simulink model "module_12s"  (R2024b)
settings: Solver=ode4  StartTime=0.0  StopTime=T_stop  FixedStep=0.1  RelTol=1e-3
settings Model: Creator=rayen  LastModifiedBy=dhia
settings DebuggingCC: AlgebraicLoopMsg=none

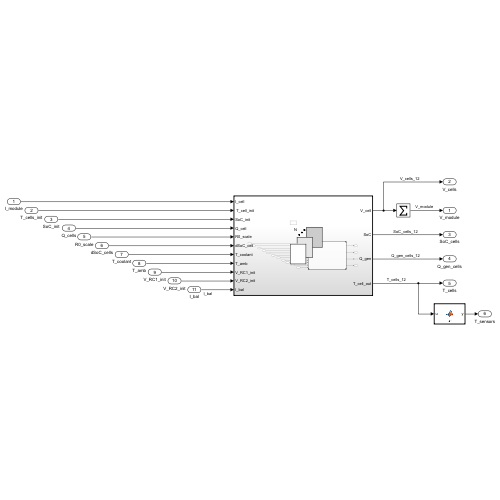
[thumbnail: Simulink's stored preview of the top-level diagram]
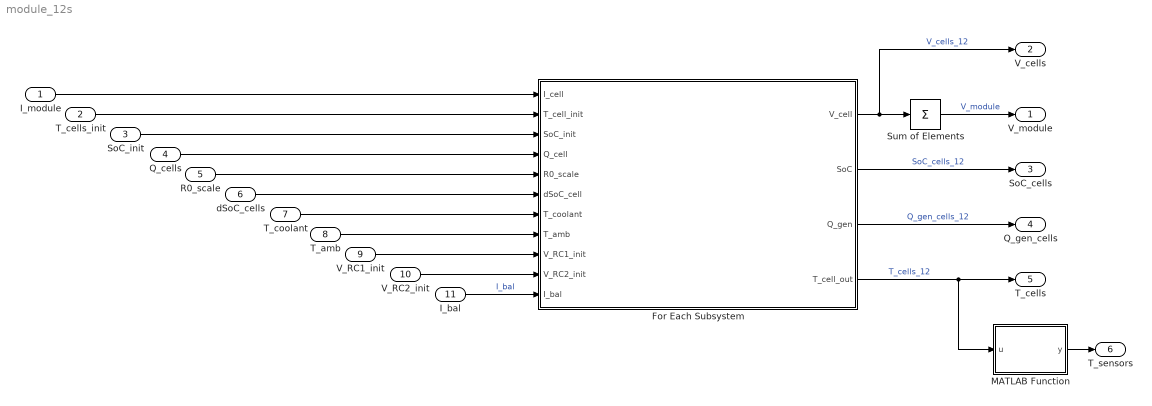
== system module_12s ==
  I_module : Inport
  T_cells_init : Inport  Port=2
  SoC_init : Inport  Port=3
  Q_cells : Inport  Port=4
  R0_scale : Inport  Port=5
  dSoC_cells : Inport  Port=6
  T_coolant : Inport  Port=7
  T_amb : Inport  Port=8
  V_RC1_init : Inport  Port=9
  V_RC2_init : Inport  Port=10
  I_bal : Inport  Port=11
  For Each Subsystem : Subsystem  TreatAsAtomicUnit=on
  MATLAB Function : MATLAB Function  TreatAsAtomicUnit=on
  Sum of Elements : Sum  Inputs=+
  V_module : Outport  PortDimensions=1
  V_cells : Outport  Port=2  PortDimensions=12
  SoC_cells : Outport  Port=3  PortDimensions=12
  Q_gen_cells : Outport  Port=4  PortDimensions=12
  T_cells : Outport  Port=5  PortDimensions=12
  T_sensors : Outport  Port=6
  wires:
  dSoC_cells/1 -> For Each Subsystem/6(dSoC_cell)
  R0_scale/1 -> For Each Subsystem/5(R0_scale)
  Q_cells/1 -> For Each Subsystem/4(Q_cell)
  SoC_init/1 -> For Each Subsystem/3(SoC_init)
  T_cells_init/1 -> For Each Subsystem/2(" T_cell_init")
  I_module/1 -> For Each Subsystem/1(I_cell)
  For Each Subsystem/1(V_cell) -> V_cells/1, Sum of Elements/1  "V_cells_12"
  Sum of Elements/1 -> V_module/1  "V_module"
  For Each Subsystem/2(SoC) -> SoC_cells/1  "SoC_cells_12"
  For Each Subsystem/3(Q_gen) -> Q_gen_cells/1  "Q_gen_cells_12"
  For Each Subsystem/4(T_cell_out) -> MATLAB Function/1(u), T_cells/1  "T_cells_12"
  T_coolant/1 -> For Each Subsystem/7(T_coolant)
  T_amb/1 -> For Each Subsystem/8(T_amb)
  V_RC1_init/1 -> For Each Subsystem/9(V_RC1_init)
  V_RC2_init/1 -> For Each Subsystem/10(V_RC2_init)
  I_bal/1 -> For Each Subsystem/11(I_bal)  "I_bal"
  MATLAB Function/1(y) -> T_sensors/1

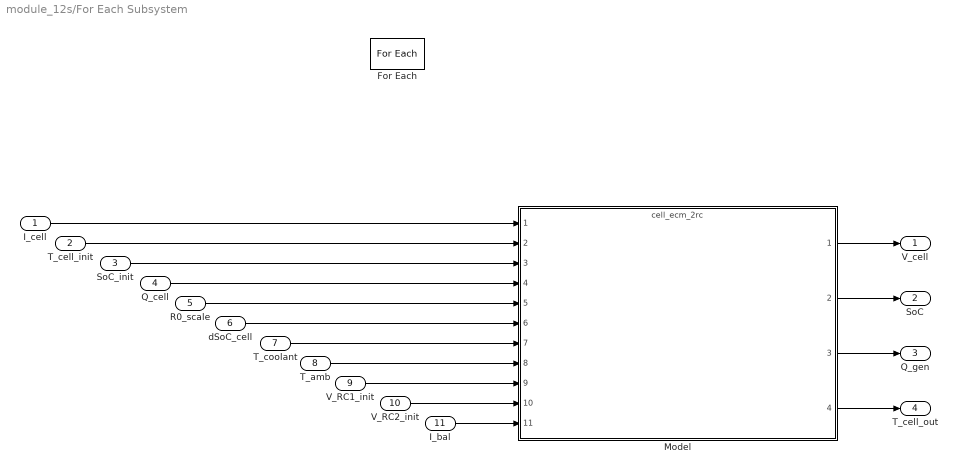
== system module_12s/For Each Subsystem ==
  I_cell : Inport
  " T_cell_init" : Inport  Port=2  Partition=on  PartitionDimension=1  PartitionWidth=1  PartitionOffset=0
  SoC_init : Inport  Port=3
  Q_cell : Inport  Port=4  Partition=on  PartitionDimension=1  PartitionWidth=1  PartitionOffset=0
  R0_scale : Inport  Port=5  Partition=on  PartitionDimension=1  PartitionWidth=1  PartitionOffset=0
  dSoC_cell : Inport  Port=6  Partition=on  PartitionDimension=1  PartitionWidth=1  PartitionOffset=0
  T_coolant : Inport  Port=7
  T_amb : Inport  Port=8
  V_RC1_init : Inport  Port=9
  V_RC2_init : Inport  Port=10
  I_bal : Inport  Port=11  Partition=on  PartitionDimension=1  PartitionWidth=1  PartitionOffset=0
  For Each : ForEach  DisableCoverage=on
  Model : ModelReference  ModelNameDialog=cell_ecm_2rc.slx  ModelReferenceVersion=1.53
  V_cell : Outport  ConcatenationDimension=1
  SoC : Outport  Port=2  ConcatenationDimension=1
  Q_gen : Outport  Port=3  ConcatenationDimension=1
  T_cell_out : Outport  Port=4  ConcatenationDimension=1
  wires:
  Model/3 -> Q_gen/1
  Model/2 -> SoC/1
  Model/1 -> V_cell/1
  I_cell/1 -> Model/1
  " T_cell_init"/1 -> Model/2
  SoC_init/1 -> Model/3
  Q_cell/1 -> Model/4
  R0_scale/1 -> Model/5
  dSoC_cell/1 -> Model/6
  Model/4 -> T_cell_out/1
  T_coolant/1 -> Model/7
  T_amb/1 -> Model/8
  V_RC1_init/1 -> Model/9
  V_RC2_init/1 -> Model/10
  I_bal/1 -> Model/11

== matlab function module_12s/MATLAB Function ==
  data: u input; y output
function y = fcn(u)

y = u;
